simulink model "Optimal_Slip_Estimator"  (R2018b)
settings: Solver=FixedStepAuto  StartTime=0.0  StopTime=10.0  RelTol=1e-3
undefined symbols (not defined in the file): OSE_Ts
settings Model: Creator=univ4123  LastModifiedBy=univ4123

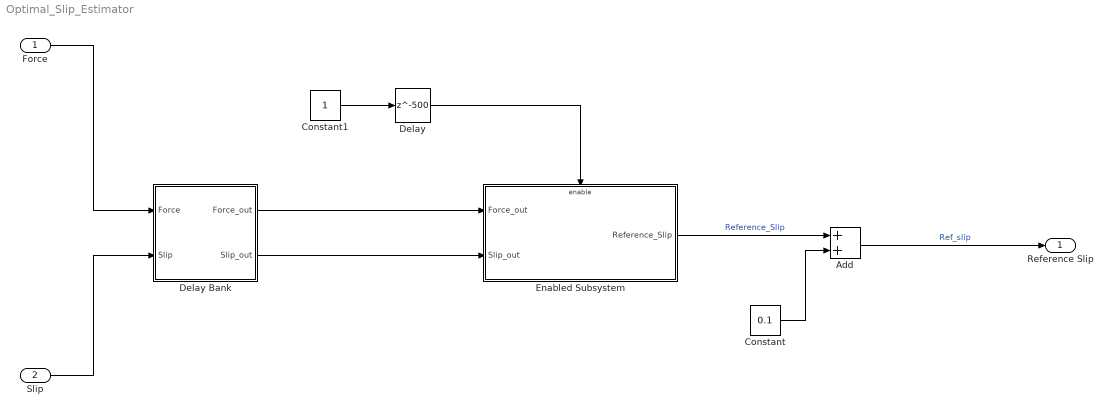
== system Optimal_Slip_Estimator ==
  "Force " : Inport
  Slip : Inport  Port=2
  Add : Sum
  Constant : Constant  Value=0.1  SampleTime=OSE_Ts
  Constant1 : Constant  SampleTime=OSE_Ts
  Delay : Delay  DelayLength=500  SampleTime=OSE_Ts
  Delay Bank : Subsystem
  Enabled Subsystem : Subsystem  TreatAsAtomicUnit=on
  Reference Slip : Outport
  wires:
  "Force "/1 -> Delay Bank/1(Force)
  Slip/1 -> Delay Bank/2("Slip ")
  Delay Bank/1(Force_out) -> Enabled Subsystem/1(Force_out)
  Delay Bank/2(Slip_out) -> Enabled Subsystem/2(Slip_out)
  Enabled Subsystem/1(Reference_Slip) -> Add/1  "Reference_Slip"
  Constant1/1 -> Delay/1
  Delay/1 -> Enabled Subsystem/Enable
  Add/1 -> Reference Slip/1  "Ref_slip"
  Constant/1 -> Add/2

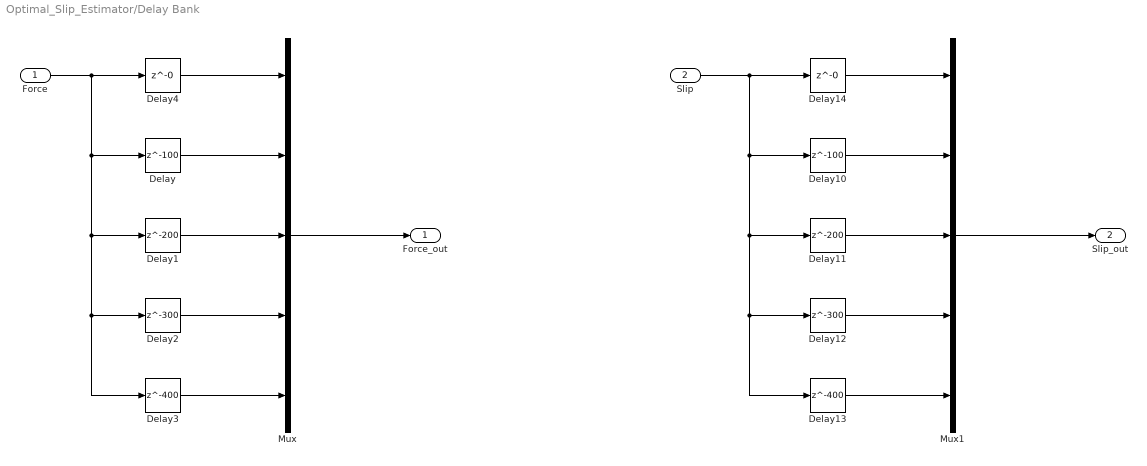
== system Optimal_Slip_Estimator/Delay Bank ==
  Force : Inport
  "Slip " : Inport  Port=2
  Delay : Delay  DelayLength=100
  Delay1 : Delay  DelayLength=200
  Delay10 : Delay  DelayLength=100
  Delay11 : Delay  DelayLength=200
  Delay12 : Delay  DelayLength=300
  Delay13 : Delay  DelayLength=400
  Delay14 : Delay  DelayLength=0
  Delay2 : Delay  DelayLength=300
  Delay3 : Delay  DelayLength=400
  Delay4 : Delay  DelayLength=0
  Mux : Mux  Inputs=5
  Mux1 : Mux  Inputs=5
  Force_out : Outport
  Slip_out : Outport  Port=2
  wires:
  Delay4/1 -> Mux/1
  Delay/1 -> Mux/2
  Delay1/1 -> Mux/3
  Delay2/1 -> Mux/4
  Delay3/1 -> Mux/5
  Delay12/1 -> Mux1/4
  Delay10/1 -> Mux1/2
  Delay14/1 -> Mux1/1
  Delay13/1 -> Mux1/5
  Delay11/1 -> Mux1/3
  "Slip "/1 -> Delay14/1, Delay10/1, Delay11/1, Delay13/1, Delay12/1
  Mux1/1 -> Slip_out/1
  Force/1 -> Delay3/1, Delay2/1, Delay1/1, Delay/1, Delay4/1
  Mux/1 -> Force_out/1

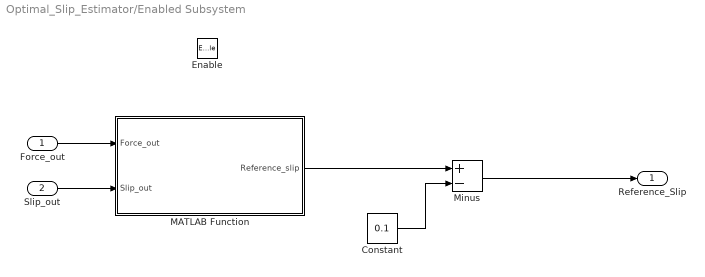
== system Optimal_Slip_Estimator/Enabled Subsystem ==
  Force_out : Inport
  Slip_out : Inport  Port=2
  Enable : EnablePort
  Constant : Constant  Value=0.1
  MATLAB Function : MATLAB Function  TreatAsAtomicUnit=on
  Minus : Sum  Inputs=+-
  Reference_Slip : Outport
  wires:
  Force_out/1 -> MATLAB Function/1(Force_out)
  Slip_out/1 -> MATLAB Function/2(Slip_out)
  MATLAB Function/1(Reference_slip) -> Minus/1
  Constant/1 -> Minus/2
  Minus/1 -> Reference_Slip/1

== matlab function Optimal_Slip_Estimator/Enabled Subsystem/MATLAB Function ==
  data: Force_out input; Reference_slip output; Slip_out input
function Reference_slip = Polyfit(Force_out, Slip_out)
%x=[0:0.01:1];
p = polyfit(Slip_out,Force_out,3);
%pcurve=polyval(p,x);
%plot(x,pcurve);

dp = polyder(p); %first derivative

d2p = polyder(dp);

m_roots=roots(dp); %roots of first derivative (max and min values)

maxmin_vals=polyval(d2p,roots(dp)); %values of the second derivative at the max and min values) (negative means maximum)

[~,I]=min(maxmin_vals); %gets which root is the maximum

Reference_slip = real(m_roots(I));
